simulink model "Simple_2Quad_payload_03"  (R2018b)
settings: Solver=VariableStepAuto  StartTime=0.0  StopTime=60  RelTol=1e-3
InitFcn:
  | Simple_2Quad_payload_03_const
values from neighbouring files (symbols this model uses):
  B = 1e0*eye(n)    [Simple_2Quad_payload_03_const.m]    (also in constant_CAMFC2_Quad_New_02_Payload_01.m = eye(n); test01.m = [eye(3) eye(3) eye(3) eye(3))
  BBT_inv = ((B'*B)^(-1))*B'    [Simple_2Quad_payload_03_const.m]    (also in Simple_4Quad_payload_04_const.m = ((BR'*BR)^(-1))*BR'; Simple_4Quad_payload_05_const.m = ((BR'*BR)^(-1))*BR'; Simple_4Quad_payload_06_const.m = ((BR'*BR)^(-1))*BR'; Simple_4Quad_payload_07_const.m = ((BR'*BR)^(-1))*BR')
  d = 1    [Simple_2Quad_payload_01_const.m]    (also in Simple_2Quad_payload_02_const.m; Simple_2Quad_payload_03_const.m; Simple_2Quad_payload_04_const.m)
  g = 9.81    [Colab_4Quad_model_01_const.m]    (also in Colab_4Quad_model_02_const.m; Simple_2Quad_payload_01_const.m; Simple_2Quad_payload_02_const.m; Simple_2Quad_payload_03_const.m)
  gamma_0 = 1e-0*diag([1e-3;1e-0])    [Simple_2Quad_payload_03_const.m]    (also in Simple_4Quad_payload_04_const.m = 1e-0*diag([1e-6*ones(3,1);1e-0*ones(3,1)]); Simple_4Quad_payload_05_const.m = 1e-1*diag([1e-6*ones(3,1);1e-0*ones(3,1)]); Simple_4Quad_payload_06_const.m = 1e-0*diag([1e-6*ones(3,1);1e-0*ones(3,1)]); Simple_4Quad_payload_07_const.m = 1e-0*diag([1e-6*ones(3,1);1e-0*ones(3,1)]))
  gamma_1 = 1e+2*diag([1e-3;1e-0])    [Simple_2Quad_payload_03_const.m]    (also in Simple_4Quad_payload_04_const.m = 1e+2*diag([1e-6*ones(3,1);1e-0*ones(3,1)]); Simple_4Quad_payload_05_const.m = 1e+2*diag([1e-6*ones(3,1);1e-0*ones(3,1)]); Simple_4Quad_payload_06_const.m = 1e+3*diag([1e-6*ones(3,1);1e-0*ones(3,1)]); Simple_4Quad_payload_07_const.m = 1e+3*diag([1e-6*ones(3,1);1e-0*ones(3,1)]))
  I = 1    [Simple_2Quad_payload_01_const.m]    (also in Simple_2Quad_payload_02_const.m; Simple_2Quad_payload_03_const.m; Simple_2Quad_payload_04_const.m)
  k1 = 1    [Simple_2Quad_payload_03_const.m]    (also in Simple_4Quad_payload_04_const.m; Simple_4Quad_payload_05_const.m; Simple_4Quad_payload_06_const.m; Simple_4Quad_payload_07_const.m)
  k2 = 0.1    [Simple_2Quad_payload_03_const.m]    (also in Simple_4Quad_payload_04_const.m; Simple_4Quad_payload_05_const.m; Simple_4Quad_payload_06_const.m; Simple_4Quad_payload_07_const.m)
  k21 = 1    [Simple_2Quad_payload_02_const.m]    (also in Simple_2Quad_payload_03_const.m)
  k22 = 1    [Simple_2Quad_payload_02_const.m]    (also in Simple_2Quad_payload_03_const.m)
  k31 = 1    [Simple_2Quad_payload_02_const.m]    (also in Simple_2Quad_payload_03_const.m)
  k32 = 1    [Simple_2Quad_payload_02_const.m]    (also in Simple_2Quad_payload_03_const.m)
  l1 = 1    [Simple_2Quad_payload_01_const.m]    (also in Simple_2Quad_payload_02_const.m; Simple_2Quad_payload_03_const.m)
  l2 = 1    [Simple_2Quad_payload_01_const.m]    (also in Simple_2Quad_payload_02_const.m; Simple_2Quad_payload_03_const.m)
  M = 1.0    (= 1)    [Colab_4Quad_model_01_const.m]    (also in Colab_4Quad_model_02_const.m; Simple_2Quad_payload_01_const.m; Simple_2Quad_payload_02_const.m; Simple_2Quad_payload_03_const.m)
  m1 = 1    [Simple_2Quad_payload_01_const.m]    (also in Simple_2Quad_payload_02_const.m; Simple_2Quad_payload_03_const.m)
  m2 = 1    [Simple_2Quad_payload_01_const.m]    (also in Simple_2Quad_payload_02_const.m; Simple_2Quad_payload_03_const.m)
  n = 2    [Simple_2Quad_payload_03_const.m]    (also in Simple_4Quad_payload_03_const.m = 6; Simple_4Quad_payload_04_const.m = 6; Simple_4Quad_payload_05_const.m = 6; Simple_4Quad_payload_06_const.m = 6)
  Q = 1e-1*eye(n)    [Simple_2Quad_payload_03_const.m]    (also in constant_CAMFC2_Quad_New_02_Payload_01.m = 1e+1*eye(n))
  R = 1e+0*eye(n)    [Simple_2Quad_payload_03_const.m]    (also in Simple_4Quad_payload_04_const.m = 1e+0*eye(m); Simple_4Quad_payload_05_const.m = 1e+0*eye(m); Simple_4Quad_payload_06_const.m; Simple_4Quad_payload_07_const.m)
  rho_0 = 1e-0    (= 1)    [Simple_2Quad_payload_03_const.m]    (also in Simple_4Quad_payload_04_const.m; Simple_4Quad_payload_05_const.m = 0.1; Simple_4Quad_payload_06_const.m; Simple_4Quad_payload_07_const.m)
  rho_1 = 1e-0    (= 1)    [Simple_2Quad_payload_03_const.m]    (also in Simple_4Quad_payload_04_const.m; Simple_4Quad_payload_05_const.m; Simple_4Quad_payload_06_const.m; Simple_4Quad_payload_07_const.m)
settings Model: Creator=ali  LastModifiedBy=ali

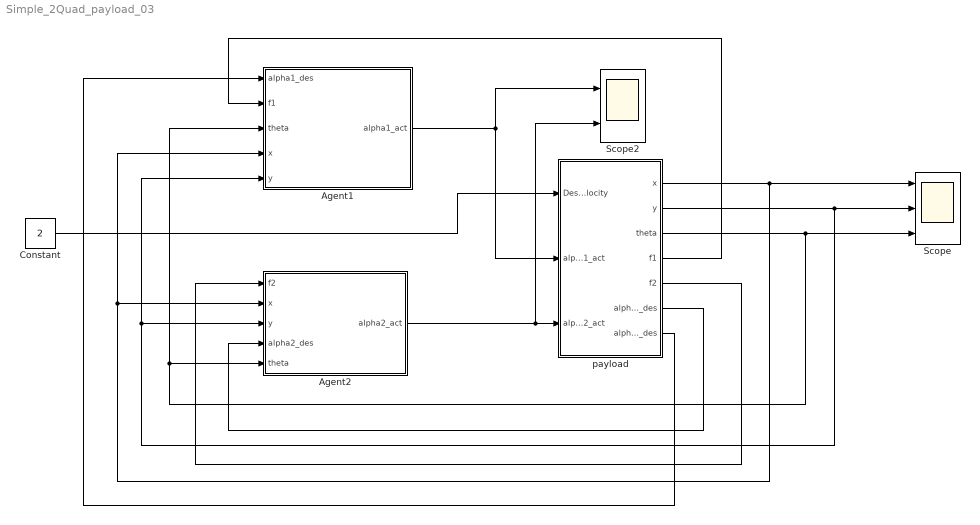
== system Simple_2Quad_payload_03 ==
  Agent1 : Subsystem
  Agent2 : Subsystem
  Constant : Constant  Value=2
  Scope : Scope  NumInputPorts=3
  Scope2 : Scope  NumInputPorts=2
  payload : Subsystem
  wires:
  Constant/1 -> payload/1(Desired_velocity)
  payload/3(theta) -> Agent2/5(theta), Agent1/3(theta), Scope/3
  payload/1(x) -> Scope/1, Agent2/2(x), Agent1/4(x)
  payload/2(y) -> Agent2/3(y), Agent1/5(y), Scope/2
  payload/4(f1) -> Agent1/2(f1)
  payload/5(f2) -> Agent2/1(f2)
  payload/6(alpha2_des) -> Agent2/4(alpha2_des)
  Agent2/1(alpha2_act) -> Scope2/2, payload/3(alpha2_act)
  Agent1/1(alpha1_act) -> Scope2/1, payload/2(alpha1_act)
  payload/7(alpha1_des) -> Agent1/1(alpha1_des)

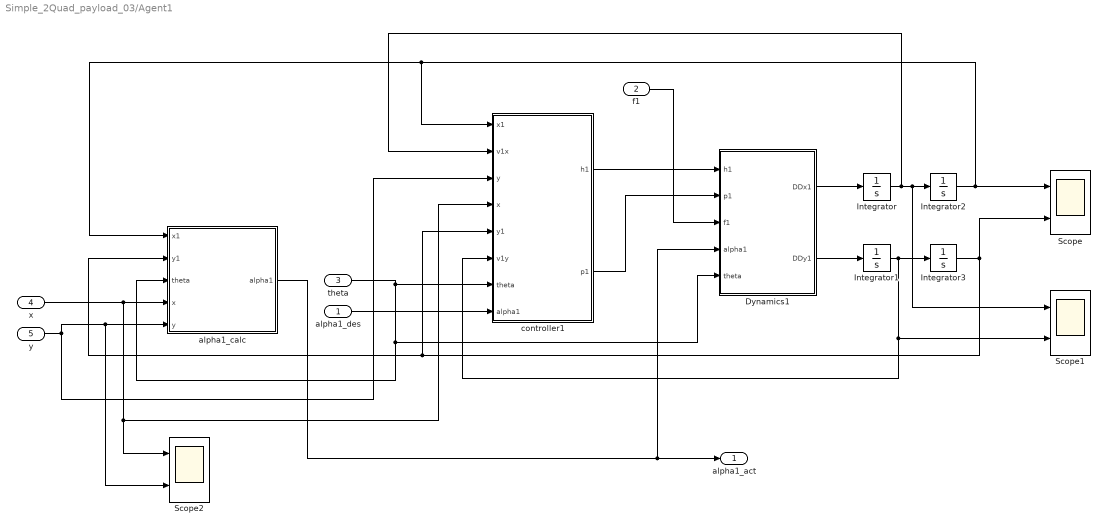
== system Simple_2Quad_payload_03/Agent1 ==
  alpha1_des : Inport
  f1 : Inport  Port=2
  theta : Inport  Port=3
  x : Inport  Port=4
  y : Inport  Port=5
  Dynamics1 : MATLAB Function  TreatAsAtomicUnit=on
  Integrator : Integrator
  Integrator1 : Integrator
  Integrator2 : Integrator  InitialCondition=1
  Integrator3 : Integrator  InitialCondition=10
  Scope : Scope  NumInputPorts=2
  Scope1 : Scope  NumInputPorts=2
  Scope2 : Scope  NumInputPorts=2
  alpha1_calc : MATLAB Function  TreatAsAtomicUnit=on
  controller1 : Subsystem
  alpha1_act : Outport
  wires:
  Dynamics1/1(DDx1) -> Integrator/1
  Dynamics1/2(DDy1) -> Integrator1/1
  Integrator/1 -> controller1/2(v1x), Scope1/1, Integrator2/1
  Integrator1/1 -> controller1/6(v1y), Scope1/2, Integrator3/1
  Integrator2/1 -> Scope/1, controller1/1(x1), alpha1_calc/1(x1)
  Integrator3/1 -> controller1/5(y1), alpha1_calc/2(y1), Scope/2
  alpha1_calc/1(alpha1) -> Dynamics1/4(alpha1), alpha1_act/1
  theta/1 -> Dynamics1/5(theta), alpha1_calc/3(theta), controller1/7(theta)
  x/1 -> Scope2/1, controller1/4(x), alpha1_calc/4(x)
  y/1 -> controller1/3(y), Scope2/2, alpha1_calc/5(y)
  controller1/2(p1) -> Dynamics1/2(p1)
  controller1/1(h1) -> Dynamics1/1(h1)
  f1/1 -> Dynamics1/3(f1)
  alpha1_des/1 -> controller1/8(alpha1)

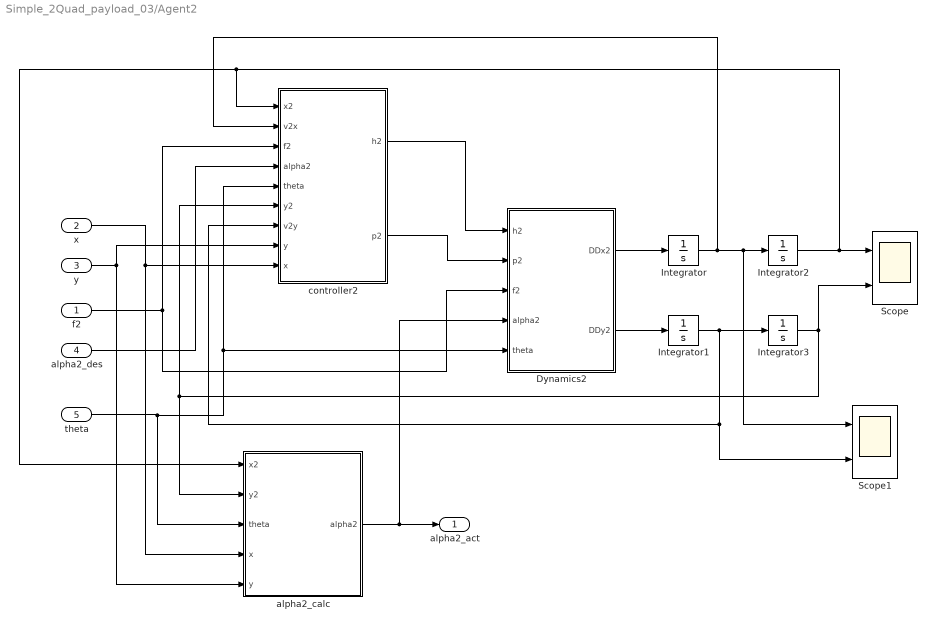
== system Simple_2Quad_payload_03/Agent2 ==
  f2 : Inport
  x : Inport  Port=2
  y : Inport  Port=3
  alpha2_des : Inport  Port=4
  theta : Inport  Port=5
  Dynamics2 : MATLAB Function  TreatAsAtomicUnit=on
  Integrator : Integrator
  Integrator1 : Integrator
  Integrator2 : Integrator  InitialCondition=-1
  Integrator3 : Integrator  InitialCondition=10
  Scope : Scope  NumInputPorts=2
  Scope1 : Scope  NumInputPorts=2
  alpha2_calc : MATLAB Function  TreatAsAtomicUnit=on
  controller2 : Subsystem
  alpha2_act : Outport
  wires:
  theta/1 -> controller2/5(theta), Dynamics2/5(theta), alpha2_calc/3(theta)
  alpha2_des/1 -> controller2/4(alpha2)
  f2/1 -> Dynamics2/3(f2), controller2/3(f2)
  controller2/1(h2) -> Dynamics2/1(h2)
  controller2/2(p2) -> Dynamics2/2(p2)
  Integrator3/1 -> alpha2_calc/2(y2), controller2/6(y2), Scope/2
  Integrator2/1 -> controller2/1(x2), alpha2_calc/1(x2), Scope/1
  Integrator1/1 -> Scope1/2, controller2/7(v2y), Integrator3/1
  Integrator/1 -> controller2/2(v2x), Scope1/1, Integrator2/1
  Dynamics2/2(DDy2) -> Integrator1/1
  Dynamics2/1(DDx2) -> Integrator/1
  y/1 -> alpha2_calc/5(y), controller2/8(y)
  x/1 -> alpha2_calc/4(x), controller2/9(x)
  alpha2_calc/1(alpha2) -> Dynamics2/4(alpha2), alpha2_act/1

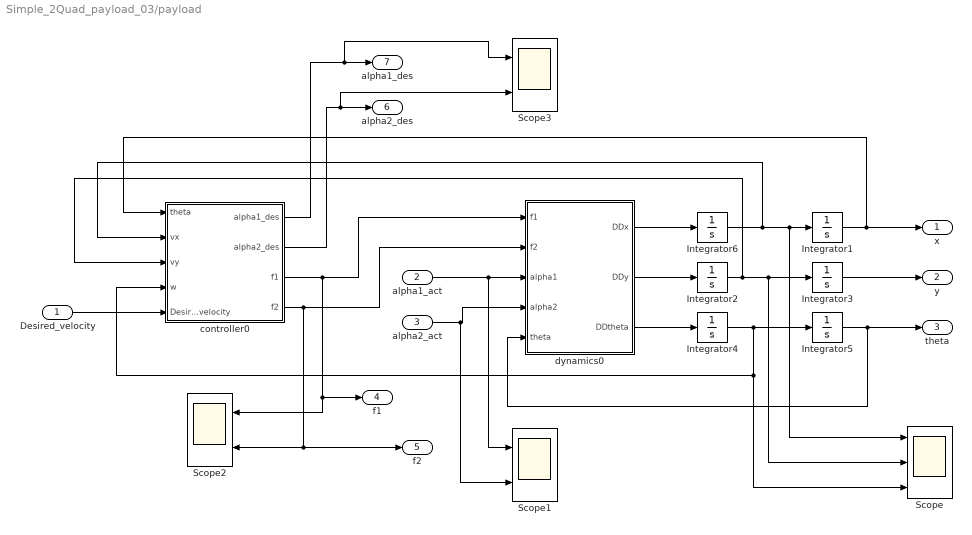
== system Simple_2Quad_payload_03/payload ==
  Desired_velocity : Inport
  alpha1_act : Inport  Port=2
  alpha2_act : Inport  Port=3
  Integrator{1..2,4..6} (5 alike) : Integrator
  Integrator3 : Integrator  InitialCondition=9
  Scope : Scope  NumInputPorts=3
  Scope1 : Scope  NumInputPorts=2
  Scope2 : Scope  NumInputPorts=2
  Scope3 : Scope  NumInputPorts=2
  controller0 : Subsystem
  dynamics0 : MATLAB Function  TreatAsAtomicUnit=on
  x : Outport
  y : Outport  Port=2
  theta : Outport  Port=3
  f1 : Outport  Port=4
  f2 : Outport  Port=5
  alpha2_des : Outport  Port=6
  alpha1_des : Outport  Port=7
  wires:
  dynamics0/1(DDx) -> Integrator6/1
  dynamics0/2(DDy) -> Integrator2/1
  dynamics0/3(DDtheta) -> Integrator4/1
  Integrator4/1 -> controller0/4(w), Scope/3, Integrator5/1
  Integrator1/1 -> controller0/1(theta), x/1
  Integrator3/1 -> y/1
  Integrator5/1 -> dynamics0/5(theta), theta/1
  Integrator2/1 -> controller0/3(vy), Scope/2, Integrator3/1
  Integrator6/1 -> controller0/2(vx), Scope/1, Integrator1/1
  Desired_velocity/1 -> controller0/5(Desired_velocity)
  controller0/3(f1) -> Scope2/1, f1/1, dynamics0/1(f1)
  controller0/4(f2) -> Scope2/2, f2/1, dynamics0/2(f2)
  controller0/1(alpha1_des) -> Scope3/1, alpha1_des/1
  controller0/2(alpha2_des) -> Scope3/2, alpha2_des/1
  alpha1_act/1 -> Scope1/1, dynamics0/3(alpha1)
  alpha2_act/1 -> Scope1/2, dynamics0/4(alpha2)

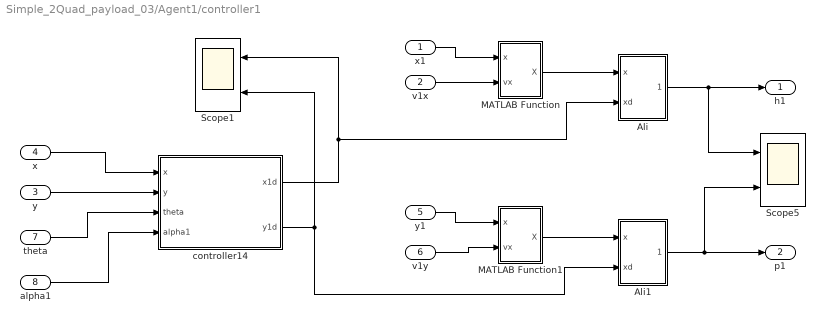
== system Simple_2Quad_payload_03/Agent1/controller1 ==
  x1 : Inport
  v1x : Inport  Port=2
  y : Inport  Port=3
  x : Inport  Port=4
  y1 : Inport  Port=5
  v1y : Inport  Port=6
  theta : Inport  Port=7
  alpha1 : Inport  Port=8
  Ali : Subsystem
  Ali1 : Subsystem
  MATLAB Function : MATLAB Function  TreatAsAtomicUnit=on
  MATLAB Function1 : MATLAB Function  TreatAsAtomicUnit=on
  Scope1 : Scope  NumInputPorts=2
  Scope5 : Scope  NumInputPorts=2
  controller14 : MATLAB Function  TreatAsAtomicUnit=on
  h1 : Outport
  p1 : Outport  Port=2
  wires:
  controller14/2(y1d) -> Ali1/2(xd), Scope1/2
  y/1 -> controller14/2(y)
  x/1 -> controller14/1(x)
  controller14/1(x1d) -> Ali/2(xd), Scope1/1
  Ali1/1(u_out) -> Scope5/2, p1/1
  Ali/1(u_out) -> Scope5/1, h1/1
  theta/1 -> controller14/3(theta)
  alpha1/1 -> controller14/4(alpha1)
  MATLAB Function/1(X) -> Ali/1(x)
  x1/1 -> MATLAB Function/1(x)
  v1x/1 -> MATLAB Function/2(vx)
  MATLAB Function1/1(X) -> Ali1/1(x)
  y1/1 -> MATLAB Function1/1(x)
  v1y/1 -> MATLAB Function1/2(vx)

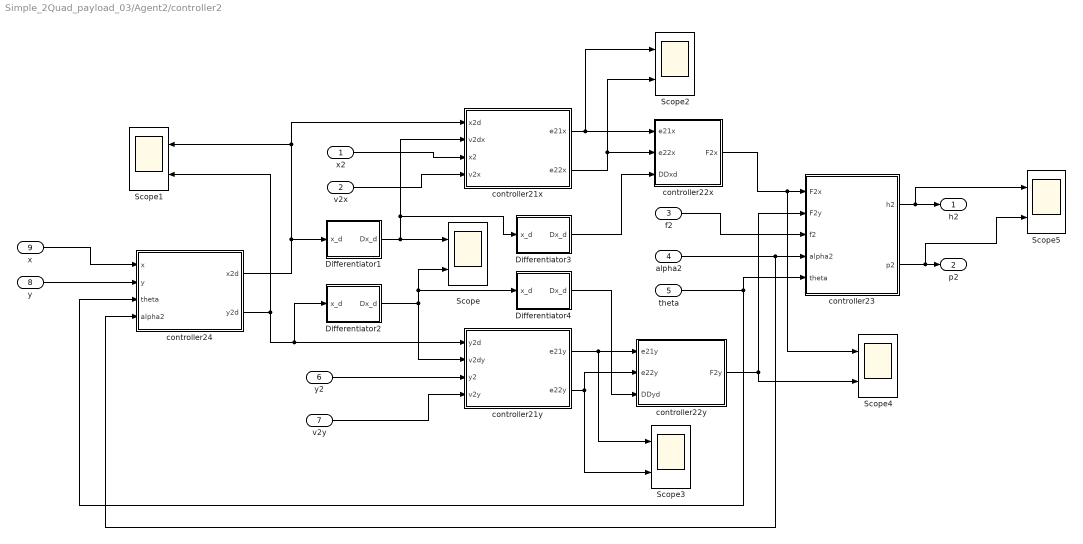
== system Simple_2Quad_payload_03/Agent2/controller2 ==
  x2 : Inport
  v2x : Inport  Port=2
  f2 : Inport  Port=3
  alpha2 : Inport  Port=4
  theta : Inport  Port=5
  y2 : Inport  Port=6
  v2y : Inport  Port=7
  y : Inport  Port=8
  x : Inport  Port=9
  Differentiator1 : Subsystem
  Differentiator2 : Subsystem
  Differentiator3 : Subsystem
  Differentiator4 : Subsystem
  Scope{,1..5} (6 alike) : Scope  NumInputPorts=2
  controller21x : MATLAB Function  TreatAsAtomicUnit=on
  controller21y : MATLAB Function  TreatAsAtomicUnit=on
  controller22x : MATLAB Function  TreatAsAtomicUnit=on
  controller22y : MATLAB Function  TreatAsAtomicUnit=on
  controller23 : MATLAB Function  TreatAsAtomicUnit=on
  controller24 : MATLAB Function  TreatAsAtomicUnit=on
  h2 : Outport
  p2 : Outport  Port=2
  wires:
  theta/1 -> controller24/3(theta), controller23/5(theta)
  alpha2/1 -> controller24/4(alpha2), controller23/4(alpha2)
  f2/1 -> controller23/3(f2)
  v2x/1 -> controller21x/4(v2x)
  x2/1 -> controller21x/3(x2)
  controller23/2(p2) -> Scope5/2, p2/1
  controller22x/1(F2x) -> Scope4/1, controller23/1(F2x)
  controller21x/1(e21x) -> Scope2/1, controller22x/1(e21x)
  controller21y/1(e21y) -> controller22y/1(e21y), Scope3/1
  controller22y/1(F2y) -> Scope4/2, controller23/2(F2y)
  y2/1 -> controller21y/3(y2)
  v2y/1 -> controller21y/4(v2y)
  controller24/1(x2d) -> Differentiator1/1(x_d), Scope1/1, controller21x/1(x2d)
  controller24/2(y2d) -> Differentiator2/1(x_d), controller21y/1(y2d), Scope1/2
  y/1 -> controller24/2(y)
  x/1 -> controller24/1(x)
  Differentiator1/1(Dx_d) -> Scope/1, Differentiator3/1(x_d), controller21x/2(v2dx)
  Differentiator2/1(Dx_d) -> Differentiator4/1(x_d), Scope/2, controller21y/2(v2dy)
  controller21x/2(e22x) -> Scope2/2, controller22x/2(e22x)
  controller21y/2(e22y) -> Scope3/2, controller22y/2(e22y)
  controller23/1(h2) -> Scope5/1, h2/1
  Differentiator3/1(Dx_d) -> controller22x/3(DDxd)
  Differentiator4/1(Dx_d) -> controller22y/3(DDyd)

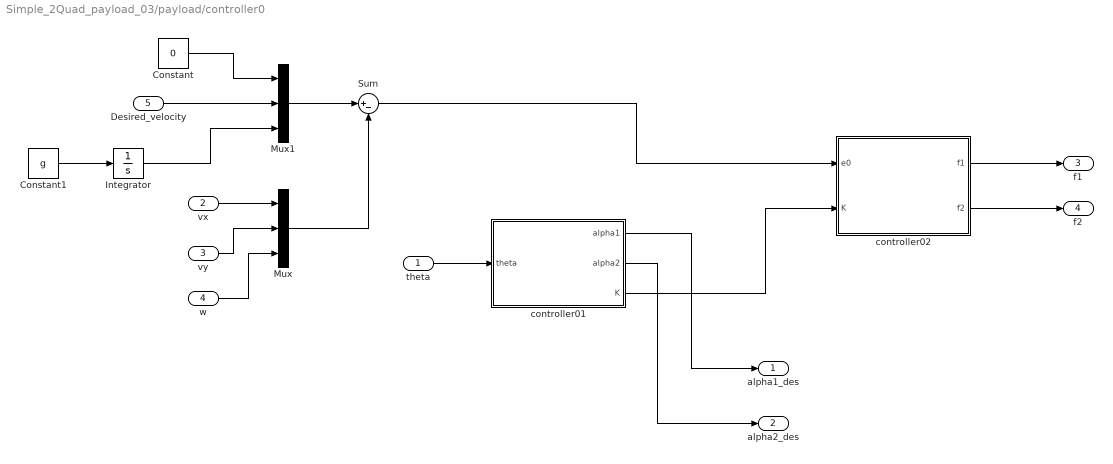
== system Simple_2Quad_payload_03/payload/controller0 ==
  theta : Inport
  vx : Inport  Port=2
  vy : Inport  Port=3
  w : Inport  Port=4
  Desired_velocity : Inport  Port=5
  Constant : Constant  Value=0
  Constant1 : Constant  Value=g
  Integrator : Integrator
  Mux : Mux  Inputs=3
  Mux1 : Mux  Inputs=3
  Sum : Sum  Inputs=|+-
  controller01 : MATLAB Function  TreatAsAtomicUnit=on
  controller02 : MATLAB Function  TreatAsAtomicUnit=on
  alpha1_des : Outport
  alpha2_des : Outport  Port=2
  f1 : Outport  Port=3
  f2 : Outport  Port=4
  wires:
  controller01/3(K) -> controller02/2(K)
  controller01/1(alpha1) -> alpha1_des/1
  controller01/2(alpha2) -> alpha2_des/1
  controller02/2(f2) -> f2/1
  controller02/1(f1) -> f1/1
  theta/1 -> controller01/1(theta)
  vx/1 -> Mux/1
  vy/1 -> Mux/2
  w/1 -> Mux/3
  Mux/1 -> Sum/2
  Sum/1 -> controller02/1(e0)
  Mux1/1 -> Sum/1
  Desired_velocity/1 -> Mux1/2
  Constant/1 -> Mux1/1
  Constant1/1 -> Integrator/1
  Integrator/1 -> Mux1/3

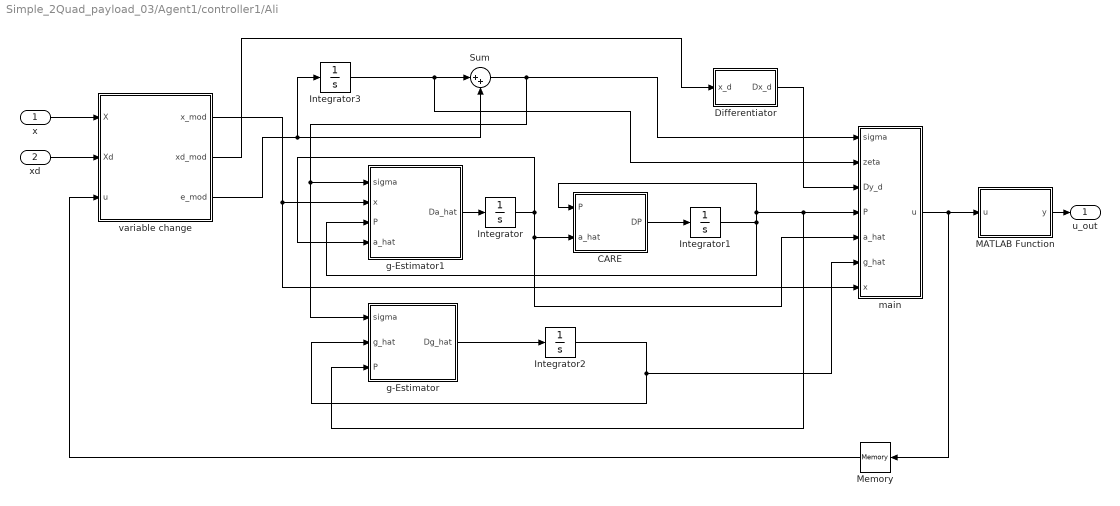
== system Simple_2Quad_payload_03/Agent1/controller1/Ali ==
  x : Inport
  xd : Inport  Port=2
  CARE : MATLAB Function  TreatAsAtomicUnit=on
  Differentiator : Subsystem
  Integrator : Integrator  InitialCondition=zeros(n)
  Integrator1 : Integrator  InitialCondition=eye(n)
  Integrator2 : Integrator  InitialCondition=zeros(n,1)
  Integrator3 : Integrator  InitialCondition=zeros(n,1)
  MATLAB Function : MATLAB Function  TreatAsAtomicUnit=on
  Memory : Memory  InitialCondition=zeros(n,1)
  Sum : Sum  Inputs=|++
  g-Estimator : MATLAB Function  TreatAsAtomicUnit=on
  g-Estimator1 : MATLAB Function  TreatAsAtomicUnit=on
  main : MATLAB Function  TreatAsAtomicUnit=on
  variable change : MATLAB Function  TreatAsAtomicUnit=on
  u_out : Outport
  wires:
  xd/1 -> variable change/2(Xd)
  x/1 -> variable change/1(X)
  Integrator/1 -> main/5(a_hat), CARE/2(a_hat), g-Estimator1/4(a_hat)
  Integrator1/1 -> g-Estimator1/3(P), main/4(P), g-Estimator/3(P), CARE/1(P)
  Sum/1 -> g-Estimator1/1(sigma), g-Estimator/1(sigma), main/1(sigma)
  Differentiator/1(Dx_d) -> main/3(Dy_d)
  g-Estimator1/1(Da_hat) -> Integrator/1
  variable change/1(x_mod) -> g-Estimator1/2(x), main/7(x)
  Integrator2/1 -> g-Estimator/2(g_hat), main/6(g_hat)
  g-Estimator/1(Dg_hat) -> Integrator2/1
  Integrator3/1 -> Sum/1, main/2(zeta)
  Memory/1 -> variable change/3(u)
  main/1(u) -> MATLAB Function/1(u), Memory/1
  CARE/1(DP) -> Integrator1/1
  variable change/2(xd_mod) -> Differentiator/1(x_d)
  variable change/3(e_mod) -> Integrator3/1, Sum/2
  MATLAB Function/1(y) -> u_out/1

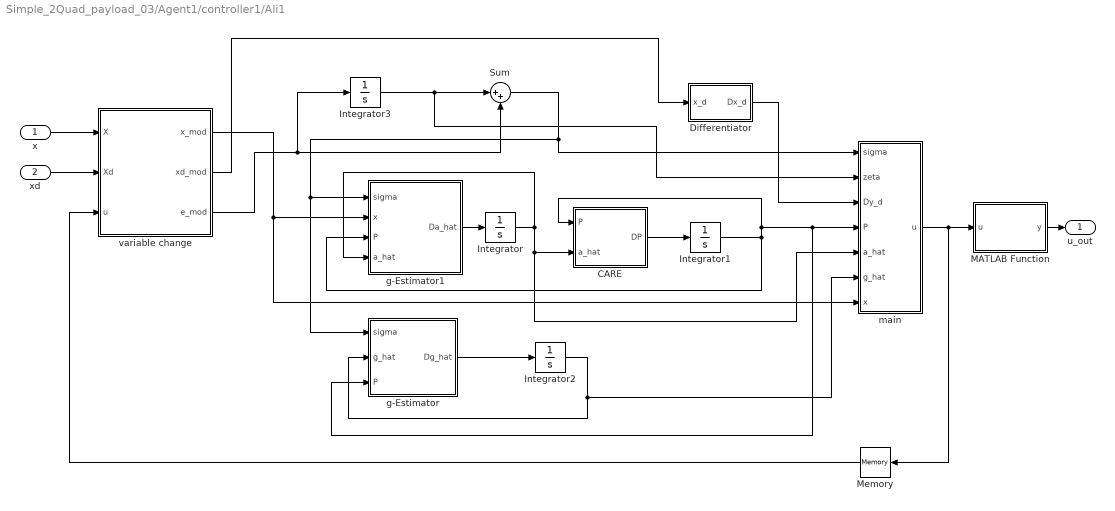
== system Simple_2Quad_payload_03/Agent1/controller1/Ali1 ==
  x : Inport
  xd : Inport  Port=2
  CARE : MATLAB Function  TreatAsAtomicUnit=on
  Differentiator : Subsystem
  Integrator : Integrator  InitialCondition=zeros(n)
  Integrator1 : Integrator  InitialCondition=eye(n)
  Integrator2 : Integrator  InitialCondition=zeros(n,1)
  Integrator3 : Integrator  InitialCondition=zeros(n,1)
  MATLAB Function : MATLAB Function  TreatAsAtomicUnit=on
  Memory : Memory  InitialCondition=zeros(n,1)
  Sum : Sum  Inputs=|++
  g-Estimator : MATLAB Function  TreatAsAtomicUnit=on
  g-Estimator1 : MATLAB Function  TreatAsAtomicUnit=on
  main : MATLAB Function  TreatAsAtomicUnit=on
  variable change : MATLAB Function  TreatAsAtomicUnit=on
  u_out : Outport
  wires:
  variable change/3(e_mod) -> Sum/2, Integrator3/1
  variable change/2(xd_mod) -> Differentiator/1(x_d)
  CARE/1(DP) -> Integrator1/1
  main/1(u) -> MATLAB Function/1(u), Memory/1
  Memory/1 -> variable change/3(u)
  Integrator3/1 -> main/2(zeta), Sum/1
  g-Estimator/1(Dg_hat) -> Integrator2/1
  Integrator2/1 -> g-Estimator/2(g_hat), main/6(g_hat)
  variable change/1(x_mod) -> main/7(x), g-Estimator1/2(x)
  g-Estimator1/1(Da_hat) -> Integrator/1
  Differentiator/1(Dx_d) -> main/3(Dy_d)
  Sum/1 -> main/1(sigma), g-Estimator/1(sigma), g-Estimator1/1(sigma)
  Integrator1/1 -> CARE/1(P), g-Estimator/3(P), main/4(P), g-Estimator1/3(P)
  Integrator/1 -> g-Estimator1/4(a_hat), CARE/2(a_hat), main/5(a_hat)
  x/1 -> variable change/1(X)
  xd/1 -> variable change/2(Xd)
  MATLAB Function/1(y) -> u_out/1

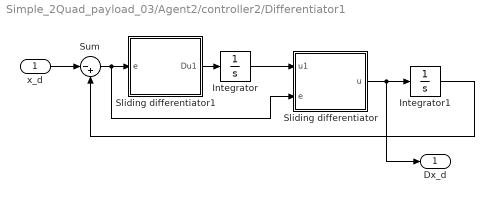
== system Simple_2Quad_payload_03/Agent2/controller2/Differentiator1 ==
  x_d : Inport
  Integrator : Integrator  InitialCondition=1
  Integrator1 : Integrator  InitialCondition=1
  Sliding differentiator : MATLAB Function  TreatAsAtomicUnit=on
  Sliding differentiator1 : MATLAB Function  TreatAsAtomicUnit=on
  Sum : Sum  Inputs=|-+
  Dx_d : Outport
  wires:
  Sliding differentiator/1(u) -> Integrator1/1, Dx_d/1
  Sliding differentiator1/1(Du1) -> Integrator/1
  Integrator/1 -> Sliding differentiator/1(u1)
  x_d/1 -> Sum/1
  Sum/1 -> Sliding differentiator/2(e), Sliding differentiator1/1(e)
  Integrator1/1 -> Sum/2

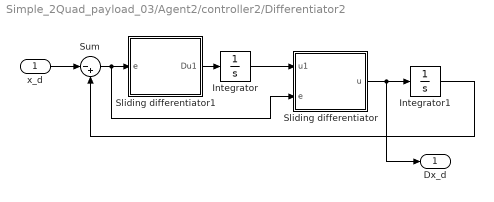
== system Simple_2Quad_payload_03/Agent2/controller2/Differentiator2 ==
  x_d : Inport
  Integrator : Integrator  InitialCondition=1
  Integrator1 : Integrator  InitialCondition=1
  Sliding differentiator : MATLAB Function  TreatAsAtomicUnit=on
  Sliding differentiator1 : MATLAB Function  TreatAsAtomicUnit=on
  Sum : Sum  Inputs=|-+
  Dx_d : Outport
  wires:
  Integrator1/1 -> Sum/2
  Sum/1 -> Sliding differentiator1/1(e), Sliding differentiator/2(e)
  x_d/1 -> Sum/1
  Integrator/1 -> Sliding differentiator/1(u1)
  Sliding differentiator1/1(Du1) -> Integrator/1
  Sliding differentiator/1(u) -> Dx_d/1, Integrator1/1

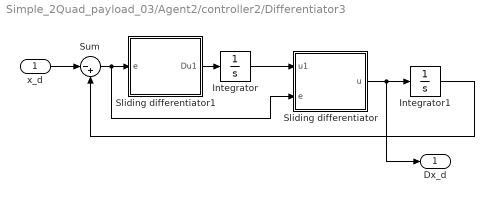
== system Simple_2Quad_payload_03/Agent2/controller2/Differentiator3 ==
  x_d : Inport
  Integrator : Integrator  InitialCondition=1
  Integrator1 : Integrator  InitialCondition=1
  Sliding differentiator : MATLAB Function  TreatAsAtomicUnit=on
  Sliding differentiator1 : MATLAB Function  TreatAsAtomicUnit=on
  Sum : Sum  Inputs=|-+
  Dx_d : Outport
  wires:
  Integrator1/1 -> Sum/2
  Sum/1 -> Sliding differentiator1/1(e), Sliding differentiator/2(e)
  x_d/1 -> Sum/1
  Integrator/1 -> Sliding differentiator/1(u1)
  Sliding differentiator1/1(Du1) -> Integrator/1
  Sliding differentiator/1(u) -> Dx_d/1, Integrator1/1

== system Simple_2Quad_payload_03/Agent2/controller2/Differentiator4 ==
  x_d : Inport
  Integrator : Integrator  InitialCondition=1
  Integrator1 : Integrator  InitialCondition=1
  Sliding differentiator : MATLAB Function  TreatAsAtomicUnit=on
  Sliding differentiator1 : MATLAB Function  TreatAsAtomicUnit=on
  Sum : Sum  Inputs=|-+
  Dx_d : Outport
  wires:
  Sliding differentiator/1(u) -> Integrator1/1, Dx_d/1
  Sliding differentiator1/1(Du1) -> Integrator/1
  Integrator/1 -> Sliding differentiator/1(u1)
  x_d/1 -> Sum/1
  Sum/1 -> Sliding differentiator/2(e), Sliding differentiator1/1(e)
  Integrator1/1 -> Sum/2

== system Simple_2Quad_payload_03/Agent1/controller1/Ali/Differentiator ==
  x_d : Inport
  Integrator : Integrator  InitialCondition=zeros(n,1)
  Integrator1 : Integrator  InitialCondition=zeros(n,1)
  Sliding differentiator : MATLAB Function  TreatAsAtomicUnit=on
  Sliding differentiator1 : MATLAB Function  TreatAsAtomicUnit=on
  Sum : Sum  Inputs=|-+
  Dx_d : Outport
  wires:
  Integrator1/1 -> Sum/2
  Sum/1 -> Sliding differentiator1/1(e), Sliding differentiator/2(e)
  x_d/1 -> Sum/1
  Integrator/1 -> Sliding differentiator/1(u1)
  Sliding differentiator1/1(Du1) -> Integrator/1
  Sliding differentiator/1(u) -> Dx_d/1, Integrator1/1

== system Simple_2Quad_payload_03/Agent1/controller1/Ali1/Differentiator ==
  x_d : Inport
  Integrator : Integrator  InitialCondition=zeros(n,1)
  Integrator1 : Integrator  InitialCondition=zeros(n,1)
  Sliding differentiator : MATLAB Function  TreatAsAtomicUnit=on
  Sliding differentiator1 : MATLAB Function  TreatAsAtomicUnit=on
  Sum : Sum  Inputs=|-+
  Dx_d : Outport
  wires:
  Sliding differentiator/1(u) -> Integrator1/1, Dx_d/1
  Sliding differentiator1/1(Du1) -> Integrator/1
  Integrator/1 -> Sliding differentiator/1(u1)
  x_d/1 -> Sum/1
  Sum/1 -> Sliding differentiator/2(e), Sliding differentiator1/1(e)
  Integrator1/1 -> Sum/2

== matlab function Simple_2Quad_payload_03/Agent1/controller1/Ali/CARE ==
  data: P input; a_hat input; B parameter; R parameter; DP output; Q parameter
function DP = fcn(P,a_hat,B,R,Q)

DP = a_hat*P + P*a_hat' - P*B*R*B'*P + 2*Q;

end

== matlab function Simple_2Quad_payload_03/Agent1/Dynamics1 ==
  data: h1 input; DDx1 output; p1 input; f1 input; alpha1 input; theta input; DDy1 output; g parameter; m1 parameter
function [DDx1,DDy1] = fcn(h1,p1,f1,alpha1,theta,g, m1)

DDx1 = (1/m1) * (h1 - f1*cos(alpha1+theta));
DDy1 = (1/m1) * (p1 - m1*g - f1*sin(alpha1+theta));

end

== matlab function Simple_2Quad_payload_03/Agent1/controller1/Ali/Differentiator/Sliding differentiator ==
  data: u output; u1 input; e input; n parameter; k1 parameter
function u = fcn(u1,e,n,k1)

b=k1;

ABS = zeros(n,1);
for i=1:n
    if e(i)>0
        ABS(i) = e(i);
    else
        ABS(i) = -e(i);
    end
end
SGN = e ./ (ABS + 0.01);

u = u1 - b*(ABS.^0.5).*SGN;

end

== matlab function Simple_2Quad_payload_03/Agent1/controller1/Ali/Differentiator/Sliding differentiator1 ==
  data: Du1 output; e input; n parameter; k2 parameter
function Du1 = fcn(e,n,k2)

a=k2;

ABS = zeros(n,1);
for i=1:n
    if e(i)>0
        ABS(i) = e(i);
    else
        ABS(i) = -e(i);
    end
end
SGN = e ./ (ABS + 0.01);

Du1 = - a*SGN;

end

== matlab function Simple_2Quad_payload_03/Agent2/Dynamics2 ==
  data: h2 input; DDx2 output; p2 input; f2 input; alpha2 input; theta input; DDy2 output; g parameter; m2 parameter
function [DDx2,DDy2] = fcn(h2,p2,f2,alpha2,theta,g, m2)

DDx2 = (1/m2) * (h2 - f2*cos(alpha2+theta));
DDy2 = (1/m2) * (p2 - m2*g - f2*sin(alpha2+theta));

end

== matlab function Simple_2Quad_payload_03/Agent2/controller2/controller22x ==
  data: e21x input; F2x output; e22x input; DDxd input
function F2x = fcn(e21x,e22x,DDxd)

k21x = 1;
k22x = 1;

F2x = DDxd + k21x*e21x + k22x*e22x;

end

== matlab function Simple_2Quad_payload_03/Agent2/controller2/controller21x ==
  data: x2d input; e21x output; v2dx input; x2 input; v2x input; e22x output
function [e21x,e22x] = fcn(x2d,v2dx,x2,v2x)

k21x = 1;

e21x = x2d - x2;
u2x = v2dx + k21x*e21x;
e22x = u2x - v2x;

end

== matlab function Simple_2Quad_payload_03/Agent2/controller2/controller23 ==
  data: F2x input; F2y input; h2 output; f2 input; alpha2 input; theta input; p2 output; m2 parameter; g parameter
function [h2,p2] = fcn(F2x,F2y,f2,alpha2,theta,m2, g)

h2 = F2x + f2*cos(alpha2+theta);
p2 = F2y + m2*g + f2*sin(alpha2+theta);

end

== matlab function Simple_2Quad_payload_03/payload/dynamics0 ==
  data: f1 input; DDx output; f2 input; alpha1 input; alpha2 input; theta input; DDy output; DDtheta output; M parameter; g parameter; d parameter; I parameter
function [DDx,DDy,DDtheta] = fcn(f1,f2,alpha1,alpha2,theta,M, g, d, I)

DDx = (1/M) * ( f1*cos(alpha1+theta) + f2*cos(alpha2+theta) );
DDy = (1/M) * ( f1*sin(alpha1+theta) + f2*sin(alpha2+theta) - M*g );
DDtheta = (d/I) * ( f1*sin(alpha1) - f2*sin(alpha2) );

end

== matlab function Simple_2Quad_payload_03/payload/controller0/controller01 ==
  data: theta input; alpha1 output; alpha2 output; k31 parameter; k22 parameter; k21 parameter; k32 parameter; K output; d parameter; M parameter; I parameter
function [alpha1,alpha2,K] = fcn(theta,k31,k22,k21, k32,d, M, I)

Kr1 = k21/k31;
Kr2 = k22/k32;

alpha1 = abs( atan( (-Kr1*sin(theta) + cos(theta)) / (Kr1*cos(theta) + sin(theta)) ) );
alpha2 = abs( atan( (-Kr2*sin(theta) + cos(theta)) / (Kr2*cos(theta) + sin(theta)) ) );

k11 = (d*M/I/k31) * (-Kr1*sin(theta) + cos(theta));
k12 = (-d*M/I/k32) * (-Kr2*sin(theta) + cos(theta));

K = [k11 k12;
    k21 k22;
    k31 k32];

end

== matlab function Simple_2Quad_payload_03/Agent1/alpha1_calc ==
  data: x1 input; alpha1 output; y1 input; theta input; d parameter; x input; y input
function alpha1 = fcn(x1,y1,theta,d, x, y)

alpha1 = ( abs( atan( (y1 - y - d*sin(theta)) / (x1 - x - d*cos(theta)) ) ) ) - theta;

end

== matlab function Simple_2Quad_payload_03/Agent2/controller2/controller21y ==
  data: y2d input; e21y output; v2dy input; y2 input; v2y input; e22y output
function [e21y,e22y] = fcn(y2d,v2dy,y2,v2y)

k21y = 1;

e21y = y2d - y2;
u2y = v2dy + k21y*e21y;
e22y = u2y - v2y;

end

== matlab function Simple_2Quad_payload_03/Agent2/controller2/controller22y ==
  data: e21y input; F2y output; e22y input; DDyd input
function F2y = fcn(e21y,e22y,DDyd)

k21y = 1;
k22y = 1;

F2y = DDyd + k21y*e21y + k22y*e22y;

end

== matlab function Simple_2Quad_payload_03/Agent2/controller2/controller24 ==
  data: x input; x2d output; y input; theta input; y2d output; alpha2 input; d parameter; l2 parameter
function [x2d,y2d] = fcn(x,y,theta,alpha2, d, l2)

x2d = x - d*cos(theta) + l2*cos(alpha2+theta);
y2d = y - d*sin(theta) + l2*sin(alpha2+theta);

end

== matlab function Simple_2Quad_payload_03/payload/controller0/controller02 ==
  data: e0 input; f1 output; D_Xd_M parameter; K input; f2 output
function [f1,f2] = fcn(e0,D_Xd_M, K)

SGN = diag(e0);
F = ((K'*K)^(-1) * K') * SGN * D_Xd_M;

f1 = F(1);
f2 = F(2);

end

== matlab function Simple_2Quad_payload_03/Agent2/alpha2_calc ==
  data: x2 input; alpha2 output; y2 input; theta input; d parameter; x input; y input
function alpha2 = fcn(x2,y2,theta,d, x, y)

alpha2 = ( abs( atan( (y2 - y + d*sin(theta)) / (x2 - x + d*cos(theta)) ) ) ) - theta;

end

== matlab function Simple_2Quad_payload_03/Agent2/controller2/Differentiator1/Sliding differentiator ==
  data: u output; u1 input; e input
function u = fcn(u1,e)

b=1;

ABS = abs(e);
SGN = e ./ (ABS + 0.01);
u = u1 - b*((ABS.^0.5).*SGN); 

end

== matlab function Simple_2Quad_payload_03/Agent2/controller2/Differentiator1/Sliding differentiator1 ==
  data: Du1 output; e input
function Du1 = fcn(e)

a=1;

ABS = abs(e);
SGN = e ./ (ABS + 0.01);
Du1 = - a*SGN;

end

== matlab function Simple_2Quad_payload_03/Agent2/controller2/Differentiator2/Sliding differentiator ==
  data: u output; u1 input; e input
function u = fcn(u1,e)

b=1;

ABS = abs(e);
SGN = e ./ (ABS + 0.01);
u = u1 - b*((ABS.^0.5).*SGN); 

end

== matlab function Simple_2Quad_payload_03/Agent2/controller2/Differentiator2/Sliding differentiator1 ==
  data: Du1 output; e input
function Du1 = fcn(e)

a=1;

ABS = abs(e);
SGN = e ./ (ABS + 0.01);
Du1 = - a*SGN;

end

== matlab function Simple_2Quad_payload_03/Agent2/controller2/Differentiator3/Sliding differentiator ==
  data: u output; u1 input; e input
function u = fcn(u1,e)

b=1;

ABS = abs(e);
SGN = e ./ (ABS + 0.01);
u = u1 - b*((ABS.^0.5).*SGN); 

end

== matlab function Simple_2Quad_payload_03/Agent2/controller2/Differentiator3/Sliding differentiator1 ==
  data: Du1 output; e input
function Du1 = fcn(e)

a=1;

ABS = abs(e);
SGN = e ./ (ABS + 0.01);
Du1 = - a*SGN;

end

== matlab function Simple_2Quad_payload_03/Agent2/controller2/Differentiator4/Sliding differentiator ==
  data: u output; u1 input; e input
function u = fcn(u1,e)

b=1;

ABS = abs(e);
SGN = e ./ (ABS + 0.01);
u = u1 - b*((ABS.^0.5).*SGN); 

end

== matlab function Simple_2Quad_payload_03/Agent2/controller2/Differentiator4/Sliding differentiator1 ==
  data: Du1 output; e input
function Du1 = fcn(e)

a=1;

ABS = abs(e);
SGN = e ./ (ABS + 0.01);
Du1 = - a*SGN;

end

== matlab function Simple_2Quad_payload_03/Agent1/controller1/Ali/g-Estimator ==
  data: sigma input; g_hat input; P input; rho_1 parameter; gamma_1 parameter; Dg_hat output
function Dg_hat = fcn(sigma,g_hat,P,rho_1,gamma_1)

Dg_hat = - gamma_1 * P * sigma - rho_1 * gamma_1 * g_hat;

end

== matlab function Simple_2Quad_payload_03/Agent1/controller1/Ali/g-Estimator1 ==
  data: sigma input; x input; P input; rho_0 parameter; gamma_0 parameter; Da_hat output; a_hat input
function Da_hat = fcn(sigma,x,P,rho_0,gamma_0,a_hat)

DVa_hat = - gamma_0 * P * diag(sigma) * (x - sigma) - rho_0 * gamma_0 * diag(a_hat);

Da_hat = diag(DVa_hat);

end

== matlab function Simple_2Quad_payload_03/Agent1/controller1/Ali/main ==
  data: sigma input; zeta input; u output; Dy_d input; R parameter; P input; a_hat input; B parameter; g_hat input; x input; Q parameter; BBT_inv parameter; n parameter
function u = fcn(sigma,zeta,Dy_d,R,P,a_hat,B,g_hat,x,Q,BBT_inv,n)

u1 = (1/2) * R * B' * P * sigma;
u2 = BBT_inv * (Dy_d - a_hat*x + (eye(n) + 2*(((P)^(-1)*Q)) + a_hat)*sigma - g_hat - zeta) - (3/4) * R * B' * P * sigma;

u = u1 + u2;

end

== matlab function Simple_2Quad_payload_03/Agent1/controller1/Ali/variable change ==
  data: X input; Xd input; x_mod output; u input; xd_mod output; e_mod output
function [x_mod,xd_mod,e_mod] = fcn(X,Xd,u)

x_mod = X;
xd_mod = [Xd;u(2)];
e_mod = xd_mod - x_mod;

end

== matlab function Simple_2Quad_payload_03/Agent1/controller1/Ali1/CARE ==
  data: P input; a_hat input; B parameter; R parameter; DP output; Q parameter
function DP = fcn(P,a_hat,B,R,Q)

DP = a_hat*P + P*a_hat' - P*B*R*B'*P + 2*Q;

end

== matlab function Simple_2Quad_payload_03/Agent1/controller1/Ali1/Differentiator/Sliding differentiator ==
  data: u output; u1 input; e input; n parameter; k1 parameter
function u = fcn(u1,e,n,k1)

b=k1;

ABS = zeros(n,1);
for i=1:n
    if e(i)>0
        ABS(i) = e(i);
    else
        ABS(i) = -e(i);
    end
end
SGN = e ./ (ABS + 0.01);

u = u1 - b*(ABS.^0.5).*SGN;

end

== matlab function Simple_2Quad_payload_03/Agent1/controller1/Ali1/Differentiator/Sliding differentiator1 ==
  data: Du1 output; e input; n parameter; k2 parameter
function Du1 = fcn(e,n,k2)

a=k2;

ABS = zeros(n,1);
for i=1:n
    if e(i)>0
        ABS(i) = e(i);
    else
        ABS(i) = -e(i);
    end
end
SGN = e ./ (ABS + 0.01);

Du1 = - a*SGN;

end

== matlab function Simple_2Quad_payload_03/Agent1/controller1/Ali1/g-Estimator ==
  data: sigma input; g_hat input; P input; rho_1 parameter; gamma_1 parameter; Dg_hat output
function Dg_hat = fcn(sigma,g_hat,P,rho_1,gamma_1)

Dg_hat = - gamma_1 * P * sigma - rho_1 * gamma_1 * g_hat;

end

== matlab function Simple_2Quad_payload_03/Agent1/controller1/Ali1/g-Estimator1 ==
  data: sigma input; x input; P input; rho_0 parameter; gamma_0 parameter; Da_hat output; a_hat input
function Da_hat = fcn(sigma,x,P,rho_0,gamma_0,a_hat)

DVa_hat = - gamma_0 * P * diag(sigma) * (x - sigma) - rho_0 * gamma_0 * diag(a_hat);

Da_hat = diag(DVa_hat);

end

== matlab function Simple_2Quad_payload_03/Agent1/controller1/MATLAB Function ==
  data: x input; X output; vx input
function X = fcn(x,vx)

X = [x;vx];

end

== matlab function Simple_2Quad_payload_03/Agent1/controller1/controller14 ==
  data: x input; x1d output; y input; theta input; y1d output; alpha1 input; d parameter; l1 parameter
function [x1d,y1d] = fcn(x,y,theta,alpha1, d, l1)

x1d = x - d*cos(theta) + l1*cos(alpha1+theta);
y1d = y - d*sin(theta) + l1*sin(alpha1+theta);

end

== matlab function Simple_2Quad_payload_03/Agent1/controller1/Ali1/main ==
  data: sigma input; zeta input; u output; Dy_d input; R parameter; P input; a_hat input; B parameter; g_hat input; x input; Q parameter; BBT_inv parameter; n parameter
function u = fcn(sigma,zeta,Dy_d,R,P,a_hat,B,g_hat,x,Q,BBT_inv,n)

u1 = (1/2) * R * B' * P * sigma;
u2 = BBT_inv * (Dy_d - a_hat*x + (eye(n) + 2*(((P)^(-1)*Q)) + a_hat)*sigma - g_hat - zeta) - (3/4) * R * B' * P * sigma;

u = u1 + u2;

end

== matlab function Simple_2Quad_payload_03/Agent1/controller1/Ali1/variable change ==
  data: X input; Xd input; x_mod output; u input; xd_mod output; e_mod output
function [x_mod,xd_mod,e_mod] = fcn(X,Xd,u)

x_mod = X;
xd_mod = [Xd;u(2)];
e_mod = xd_mod - x_mod;

end

== matlab function Simple_2Quad_payload_03/Agent1/controller1/Ali/MATLAB Function ==
  data: u input; y output
function y = fcn(u)

y = u(1);

end

== matlab function Simple_2Quad_payload_03/Agent1/controller1/Ali1/MATLAB Function ==
  data: u input; y output
function y = fcn(u)

y = u(1);

end

== matlab function Simple_2Quad_payload_03/Agent1/controller1/MATLAB Function1 ==
  data: x input; X output; vx input
function X = fcn(x,vx)

X = [x;vx];

end
